simulink model "sus"  (Simulink 6.5)
settings: Solver=ode45  StartTime=0.0  StopTime=16  RelTol=1e-3
libraries: cdsFilt x266, cdsBitwise x92, cdsEpicsOut x84, cdsEpicsBinIn x56, cdsEpicsIn x20, cdsFiltCtrl x18, cdsMatrix x11, cdsSwitch x7, cdsWD x7, cdsFunctionCall x5, cdsRio1 x4, dac x3
(part 19 of 20)

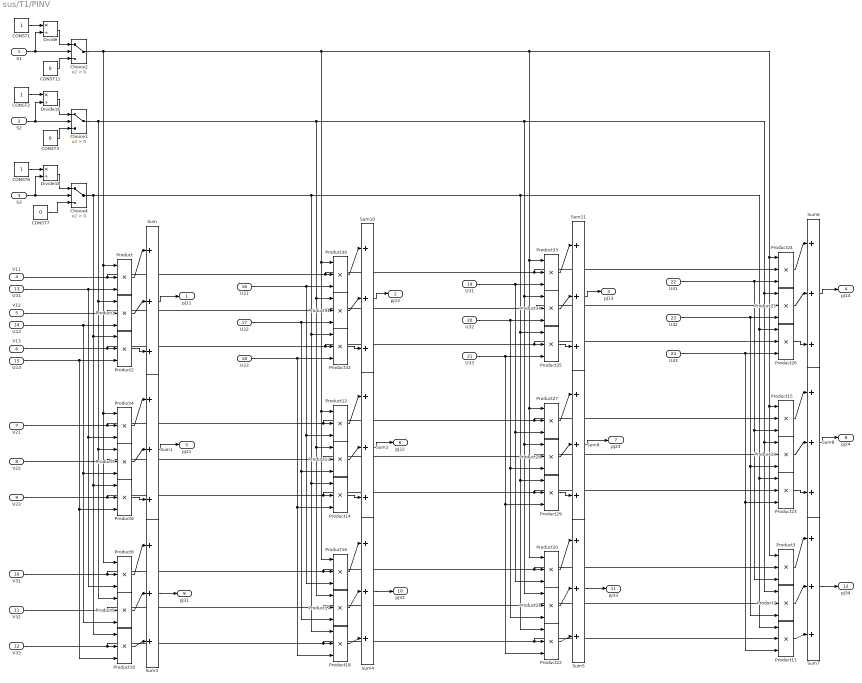
== system sus/T1/PINV ==
  S1 : Inport
  S2 : Inport  Port=2
  S3 : Inport  Port=3
  V11 : Inport  Port=4
  V12 : Inport  Port=5
  V13 : Inport  Port=6
  V21 : Inport  Port=7
  V22 : Inport  Port=8
  V23 : Inport  Port=9
  V31 : Inport  Port=10
  V32 : Inport  Port=11
  V33 : Inport  Port=12
  U11 : Inport  Port=13
  U12 : Inport  Port=14
  U13 : Inport  Port=15
  U21 : Inport  Port=16
  U22 : Inport  Port=17
  U23 : Inport  Port=18
  U31 : Inport  Port=19
  U32 : Inport  Port=20
  U33 : Inport  Port=21
  U41 : Inport  Port=22
  U42 : Inport  Port=23
  U43 : Inport  Port=24
  CONST1 : Constant
  CONST11 : Constant  Value=0
  CONST2 : Constant
  CONST3 : Constant  Value=0
  CONST6 : Constant
  CONST7 : Constant  Value=0
  Choice1 : Switch  Criteria=u2 > Threshold
  Choice2 : Switch  Criteria=u2 > Threshold
  Choice4 : Switch  Criteria=u2 > Threshold
  Divide : Product  Inputs=*/  OutScaling=2^-10
  Divide16 : Product  Inputs=*/  OutScaling=2^-10
  Divide18 : Product  Inputs=*/  OutScaling=2^-10
  Product{,1..35} (36 alike) : Product  Inputs=3  RndMeth=Zero
  Sum{,1..11} (12 alike) : Sum  Inputs=|+++
  pJ11 : Outport
  pJ12 : Outport  Port=2
  pJ13 : Outport  Port=3
  pJ14 : Outport  Port=4
  pJ21 : Outport  Port=5
  pJ22 : Outport  Port=6
  pJ23 : Outport  Port=7
  pJ24 : Outport  Port=8
  pJ31 : Outport  Port=9
  pJ32 : Outport  Port=10
  pJ33 : Outport  Port=11
  pJ34 : Outport  Port=12
  wires:
  Product/1 -> Sum/1
  S1/1 -> Choice2/2, Divide/2
  Divide/1 -> Choice2/1
  CONST11/1 -> Choice2/3
  CONST1/1 -> Divide/1
  Divide16/1 -> Choice1/1
  CONST3/1 -> Choice1/3
  CONST2/1 -> Divide16/1
  S2/1 -> Choice1/2, Divide16/2
  Divide18/1 -> Choice4/1
  CONST7/1 -> Choice4/3
  CONST6/1 -> Divide18/1
  S3/1 -> Choice4/2, Divide18/2
  Product1/1 -> Sum/2
  Product2/1 -> Sum/3
  Product4/1 -> Sum1/1
  Product5/1 -> Sum1/2
  Product6/1 -> Sum1/3
  Product8/1 -> Sum3/1
  Product9/1 -> Sum3/2
  Product10/1 -> Sum3/3
  Product30/1 -> Sum10/1
  Product31/1 -> Sum10/2
  Product32/1 -> Sum10/3
  Product12/1 -> Sum2/1
  Product13/1 -> Sum2/2
  Product14/1 -> Sum2/3
  Product16/1 -> Sum4/1
  Product17/1 -> Sum4/2
  Product18/1 -> Sum4/3
  Product33/1 -> Sum11/1
  Product34/1 -> Sum11/2
  Product35/1 -> Sum11/3
  Product27/1 -> Sum9/1
  Product28/1 -> Sum9/2
  Product29/1 -> Sum9/3
  Product20/1 -> Sum5/1
  Product21/1 -> Sum5/2
  Product22/1 -> Sum5/3
  Product24/1 -> Sum6/1
  Product25/1 -> Sum6/2
  Product26/1 -> Sum6/3
  Product15/1 -> Sum8/1
  Product19/1 -> Sum8/2
  Product23/1 -> Sum8/3
  Product3/1 -> Sum7/1
  Product7/1 -> Sum7/2
  Product11/1 -> Sum7/3
  Choice2/1 -> Product/1, Product4/1, Product8/1, Product33/1, Product20/1, Product27/1, Product24/1, Product3/1, Product15/1, Product30/1, Product12/1, Product16/1
  Choice1/1 -> Product1/1, Product5/1, Product9/1, Product34/1, Product21/1, Product28/1, Product25/1, Product7/1, Product19/1, Product31/1, Product17/1, Product13/1
  Choice4/1 -> Product2/1, Product6/1, Product10/1, Product35/1, Product22/1, Product29/1, Product26/1, Product11/1, Product23/1, Product32/1, Product18/1, Product14/1
  V11/1 -> Product/2, Product30/2, Product33/2, Product24/2
  U11/1 -> Product/3, Product4/3, Product8/3
  V12/1 -> Product1/2, Product31/2, Product34/2, Product25/2
  U12/1 -> Product1/3, Product5/3, Product9/3
  V13/1 -> Product2/2, Product32/2, Product35/2, Product26/2
  U13/1 -> Product2/3, Product6/3, Product10/3
  V21/1 -> Product4/2, Product12/2, Product27/2, Product15/2
  V22/1 -> Product5/2, Product13/2, Product28/2, Product19/2
  V23/1 -> Product6/2, Product14/2, Product29/2, Product23/2
  V31/1 -> Product8/2, Product16/2, Product20/2, Product3/2
  V32/1 -> Product9/2, Product17/2, Product21/2, Product7/2
  V33/1 -> Product10/2, Product18/2, Product22/2, Product11/2
  Sum/1 -> pJ11/1
  Sum1/1 -> pJ21/1
  Sum3/1 -> pJ31/1
  Sum10/1 -> pJ12/1
  Sum11/1 -> pJ13/1
  Sum6/1 -> pJ14/1
  Sum2/1 -> pJ22/1
  Sum9/1 -> pJ23/1
  Sum8/1 -> pJ24/1
  Sum4/1 -> pJ32/1
  Sum5/1 -> pJ33/1
  Sum7/1 -> pJ34/1
  U21/1 -> Product30/3, Product12/3, Product16/3
  U22/1 -> Product31/3, Product17/3, Product13/3
  U23/1 -> Product32/3, Product18/3, Product14/3
  U31/1 -> Product33/3, Product20/3, Product27/3
  U32/1 -> Product34/3, Product21/3, Product28/3
  U33/1 -> Product35/3, Product22/3, Product29/3
  U41/1 -> Product24/3, Product3/3, Product15/3
  U42/1 -> Product25/3, Product7/3, Product19/3
  U43/1 -> Product26/3, Product11/3, Product23/3

== system sus/T1/SQ1 ==
  11 : Inport
  12 : Inport  Port=2
  13 : Inport  Port=3
  21 : Inport  Port=4
  22 : Inport  Port=5
  23 : Inport  Port=6
  31 : Inport  Port=7
  32 : Inport  Port=8
  33 : Inport  Port=9
  41 : Inport  Port=10
  42 : Inport  Port=11
  43 : Inport  Port=12
  Product{,1..23} (24 alike) : Product  RndMeth=Zero
  Sum{,1..5} (6 alike) : Sum  Inputs=|++++
  Out11 : Outport
  Out12 : Outport  Port=2
  Out13 : Outport  Port=3
  Out21 : Outport  Port=4
  Out22 : Outport  Port=5
  Out23 : Outport  Port=6
  Out31 : Outport  Port=7
  Out32 : Outport  Port=8
  Out33 : Outport  Port=9
  wires:
  Product/1 -> Sum/1
  11/1 -> Product/1, Product/2, Product4/1, Product8/1
  Sum/1 -> Out11/1
  Product1/1 -> Sum/2
  Product2/1 -> Sum/3
  Product3/1 -> Sum/4
  21/1 -> Product1/1, Product1/2, Product5/1, Product9/1
  31/1 -> Product2/1, Product2/2, Product6/1, Product10/1
  41/1 -> Product3/1, Product3/2, Product7/1, Product11/1
  Product4/1 -> Sum1/1
  Product5/1 -> Sum1/2
  Product6/1 -> Sum1/3
  Product7/1 -> Sum1/4
  Sum1/1 -> Out21/1, Out12/1
  12/1 -> Product4/2, Product12/2, Product12/1, Product16/1
  22/1 -> Product5/2, Product13/2, Product13/1, Product17/1
  32/1 -> Product6/2, Product14/2, Product14/1, Product18/1
  42/1 -> Product7/2, Product15/2, Product15/1, Product19/1
  Product8/1 -> Sum2/1
  Product9/1 -> Sum2/2
  Product10/1 -> Sum2/3
  Product11/1 -> Sum2/4
  43/1 -> Product11/2, Product19/2, Product23/2, Product23/1
  33/1 -> Product10/2, Product18/2, Product22/2, Product22/1
  23/1 -> Product9/2, Product17/2, Product21/2, Product21/1
  13/1 -> Product8/2, Product16/2, Product20/2, Product20/1
  Sum2/1 -> Out31/1, Out13/1
  Product12/1 -> Sum3/1
  Product13/1 -> Sum3/2
  Product14/1 -> Sum3/3
  Product15/1 -> Sum3/4
  Sum3/1 -> Out22/1
  Product16/1 -> Sum4/1
  Product17/1 -> Sum4/2
  Product18/1 -> Sum4/3
  Product19/1 -> Sum4/4
  Sum4/1 -> Out32/1, Out23/1
  Product20/1 -> Sum5/1
  Product21/1 -> Sum5/2
  Product22/1 -> Sum5/3
  Product23/1 -> Sum5/4
  Sum5/1 -> Out33/1

== system sus/T1/SQRT_BOX ==
  In1 : Inport
  CONST11 : Constant  Value=0
  Choice : Switch  Threshold=1000
  Choice1 : Switch
  Choice2 : Switch  Threshold=1e10
  Choice3 : Switch  Threshold=0.01
  Choice4 : Switch  Threshold=1e-6
  Divide{,1..9} (10 alike) : Product  Inputs=*/  OutScaling=2^-10
  Gain : Gain  Gain=0.05
  Gain{1..10} (10 alike) : Gain  Gain=0.5
  Gain11 : Gain  Gain=0.0001
  Gain12 : Gain  Gain=0.000001
  Gain13 : Gain  Gain=100
  Gain14 : Gain  Gain=10000
  Sum{,1..9} (10 alike) : Sum  Inputs=|++
  Out1 : Outport
  wires:
  Divide/1 -> Sum/1
  Choice1/1 -> Choice/2, Choice2/2, Choice3/2, Choice4/2, Gain/1, Gain13/1, Gain14/1, Divide/1, Divide1/1, Divide2/1, Divide3/1, Divide4/1, Divide5/1, Divide6/1, Divide7/1, Divide8/1, Divide9/1, Gain12/1, Gain11/1
  Gain1/1 -> Sum1/2, Divide1/2
  Divide1/1 -> Sum1/1
  Sum1/1 -> Gain2/1
  Sum/1 -> Gain1/1
  Gain2/1 -> Sum2/2, Divide2/2
  Divide2/1 -> Sum2/1
  Sum2/1 -> Gain4/1
  Gain4/1 -> Sum3/2, Divide3/2
  Divide3/1 -> Sum3/1
  Sum3/1 -> Gain3/1
  Gain3/1 -> Sum4/2, Divide4/2
  Divide4/1 -> Sum4/1
  Sum4/1 -> Gain5/1
  Gain5/1 -> Sum5/2, Divide5/2
  Divide5/1 -> Sum5/1
  Sum5/1 -> Gain6/1
  Gain6/1 -> Sum6/2, Divide6/2
  Divide6/1 -> Sum6/1
  Sum6/1 -> Gain7/1
  Gain7/1 -> Sum7/2, Divide7/2
  Divide7/1 -> Sum7/1
  Sum7/1 -> Gain8/1
  Gain8/1 -> Sum8/2, Divide8/2
  Divide8/1 -> Sum8/1
  Sum8/1 -> Gain9/1
  Gain9/1 -> Sum9/2, Divide9/2
  Divide9/1 -> Sum9/1
  Sum9/1 -> Gain10/1
  Gain10/1 -> Out1/1
  Gain/1 -> Choice/3
  In1/1 -> Choice1/2, Choice1/1
  CONST11/1 -> Choice1/3
  Gain11/1 -> Choice2/3
  Gain12/1 -> Choice2/1
  Choice2/1 -> Choice/1
  Choice/1 -> Choice3/1
  Choice3/1 -> Choice4/1
  Choice4/1 -> Sum/2, Divide/2
  Gain13/1 -> Choice3/3
  Gain14/1 -> Choice4/3

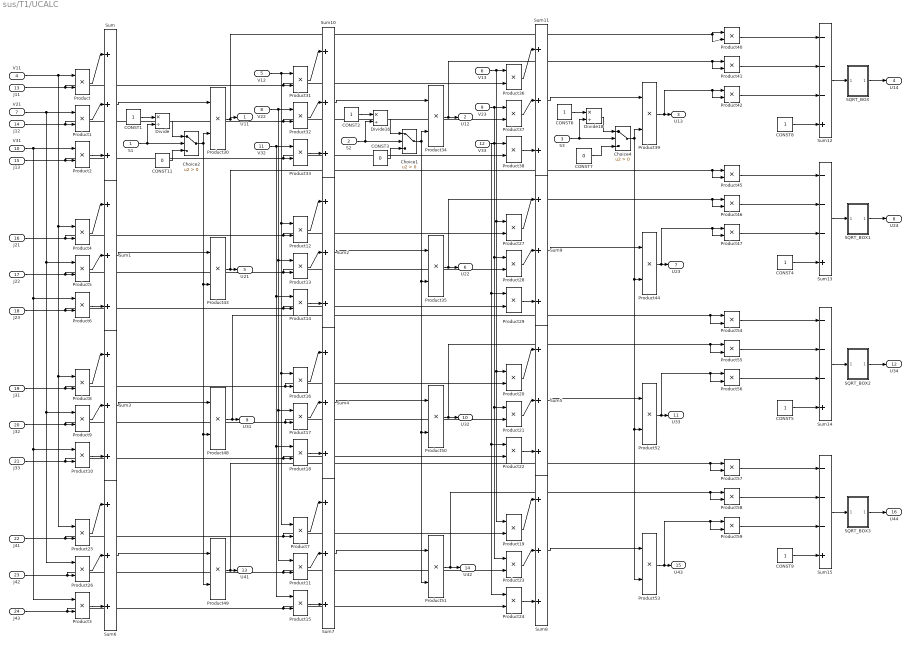
== system sus/T1/UCALC ==
  S1 : Inport
  S2 : Inport  Port=2
  S3 : Inport  Port=3
  V11 : Inport  Port=4
  V12 : Inport  Port=5
  V13 : Inport  Port=6
  V21 : Inport  Port=7
  V22 : Inport  Port=8
  V23 : Inport  Port=9
  V31 : Inport  Port=10
  V32 : Inport  Port=11
  V33 : Inport  Port=12
  J11 : Inport  Port=13
  J12 : Inport  Port=14
  J13 : Inport  Port=15
  J21 : Inport  Port=16
  J22 : Inport  Port=17
  J23 : Inport  Port=18
  J31 : Inport  Port=19
  J32 : Inport  Port=20
  J33 : Inport  Port=21
  J41 : Inport  Port=22
  J42 : Inport  Port=23
  J43 : Inport  Port=24
  CONST{1..2,4..6,8..9} (7 alike) : Constant
  CONST11 : Constant  Value=0
  CONST3 : Constant  Value=0
  CONST7 : Constant  Value=0
  Choice1 : Switch  Criteria=u2 > Threshold
  Choice2 : Switch  Criteria=u2 > Threshold
  Choice4 : Switch  Criteria=u2 > Threshold
  Divide : Product  Inputs=*/  OutScaling=2^-10
  Divide16 : Product  Inputs=*/  OutScaling=2^-10
  Divide18 : Product  Inputs=*/  OutScaling=2^-10
  Product{,1..59} (60 alike) : Product  RndMeth=Zero
  SQRT_BOX : Subsystem
  SQRT_BOX1 : Subsystem
  SQRT_BOX2 : Subsystem
  SQRT_BOX3 : Subsystem
  Sum{,1..11} (12 alike) : Sum  Inputs=|+++
  Sum{12..15} (4 alike) : Sum  Inputs=---+
  U11 : Outport
  U12 : Outport  Port=2
  U13 : Outport  Port=3
  U14 : Outport  Port=4
  U21 : Outport  Port=5
  U22 : Outport  Port=6
  U23 : Outport  Port=7
  U24 : Outport  Port=8
  U31 : Outport  Port=9
  U32 : Outport  Port=10
  U33 : Outport  Port=11
  U34 : Outport  Port=12
  U41 : Outport  Port=13
  U42 : Outport  Port=14
  U43 : Outport  Port=15
  U44 : Outport  Port=16
  wires:
  Product20/1 -> Sum5/1
  Product21/1 -> Sum5/2
  Product22/1 -> Sum5/3
  Product19/1 -> Sum8/1
  Product23/1 -> Sum8/2
  Product24/1 -> Sum8/3
  Product12/1 -> Sum2/1
  Product13/1 -> Sum2/2
  Product14/1 -> Sum2/3
  Product16/1 -> Sum4/1
  Product17/1 -> Sum4/2
  Product18/1 -> Sum4/3
  Product7/1 -> Sum7/1
  Product11/1 -> Sum7/2
  Product15/1 -> Sum7/3
  Product/1 -> Sum/1
  Product1/1 -> Sum/2
  Product2/1 -> Sum/3
  Product4/1 -> Sum1/1
  Product5/1 -> Sum1/2
  Product6/1 -> Sum1/3
  Product8/1 -> Sum3/1
  Product9/1 -> Sum3/2
  Product10/1 -> Sum3/3
  Product25/1 -> Sum6/1
  Product26/1 -> Sum6/2
  Product3/1 -> Sum6/3
  V11/1 -> Product/1, Product4/1, Product8/1, Product25/1
  J11/1 -> Product/2, Product31/2, Product36/2
  V21/1 -> Product1/1, Product5/1, Product9/1, Product26/1
  J12/1 -> Product1/2, Product32/2, Product37/2
  J13/1 -> Product2/2, Product33/2, Product38/2
  V31/1 -> Product2/1, Product6/1, Product10/1, Product3/1
  S1/1 -> Choice2/2, Divide/2
  Divide/1 -> Choice2/1
  CONST11/1 -> Choice2/3
  CONST1/1 -> Divide/1
  Product30/1 -> U11/1, Product40/1, Product40/2
  Choice2/1 -> Product30/2, Product43/2, Product48/2, Product49/2
  Sum/1 -> Product30/1
  Product31/1 -> Sum10/1
  Product32/1 -> Sum10/2
  Product33/1 -> Sum10/3
  V12/1 -> Product31/1, Product12/1, Product16/1, Product7/1
  V22/1 -> Product32/1, Product13/1, Product17/1, Product11/1
  V32/1 -> Product33/1, Product14/1, Product18/1, Product15/1
  Divide16/1 -> Choice1/1
  CONST3/1 -> Choice1/3
  CONST2/1 -> Divide16/1
  Choice1/1 -> Product34/2, Product35/2, Product50/2, Product51/2
  Sum10/1 -> Product34/1
  S2/1 -> Choice1/2, Divide16/2
  Product34/1 -> U12/1, Product41/1, Product41/2
  Product36/1 -> Sum11/1
  Product37/1 -> Sum11/2
  Product38/1 -> Sum11/3
  V13/1 -> Product36/1, Product27/1, Product20/1, Product19/1
  V23/1 -> Product37/1, Product28/1, Product21/1, Product23/1
  V33/1 -> Product38/1, Product29/1, Product22/1, Product24/1
  Divide18/1 -> Choice4/1
  CONST7/1 -> Choice4/3
  CONST6/1 -> Divide18/1
  Choice4/1 -> Product39/2, Product44/2, Product52/2, Product53/2
  Sum11/1 -> Product39/1
  S3/1 -> Choice4/2, Divide18/2
  Product39/1 -> U13/1, Product42/1, Product42/2
  J21/1 -> Product4/2, Product12/2, Product27/2
  J22/1 -> Product5/2, Product13/2, Product28/2
  J23/1 -> Product6/2, Product14/2, Product29/2
  J31/1 -> Product8/2, Product16/2, Product20/2
  J32/1 -> Product9/2, Product17/2, Product21/2
  J33/1 -> Product10/2, Product18/2, Product22/2
  J41/1 -> Product25/2, Product7/2, Product19/2
  J42/1 -> Product26/2, Product11/2, Product23/2
  J43/1 -> Product3/2, Product15/2, Product24/2
  CONST8/1 -> Sum12/4
  Product40/1 -> Sum12/1
  Product41/1 -> Sum12/2
  Product42/1 -> Sum12/3
  Sum12/1 -> SQRT_BOX/1(In1)
  SQRT_BOX/1(Out1) -> U14/1
  Product27/1 -> Sum9/1
  Product28/1 -> Sum9/2
  Sum1/1 -> Product43/1
  Product43/1 -> U21/1, Product45/1, Product45/2
  Sum2/1 -> Product35/1
  Product35/1 -> U22/1, Product46/1, Product46/2
  Sum9/1 -> Product44/1
  Product44/1 -> U23/1, Product47/1, Product47/2
  CONST4/1 -> Sum13/4
  Product45/1 -> Sum13/1
  Product46/1 -> Sum13/2
  Product47/1 -> Sum13/3
  Sum13/1 -> SQRT_BOX1/1(In1)
  SQRT_BOX1/1(Out1) -> U24/1
  Sum3/1 -> Product48/1
  Product48/1 -> U31/1, Product54/1, Product54/2
  Sum6/1 -> Product49/1
  Product49/1 -> U41/1, Product57/1, Product57/2
  Product50/1 -> U32/1, Product55/1, Product55/2
  Product51/1 -> U42/1, Product58/1, Product58/2
  Sum4/1 -> Product50/1
  Sum7/1 -> Product51/1
  Sum5/1 -> Product52/1
  Product52/1 -> U33/1, Product56/1, Product56/2
  Product53/1 -> U43/1, Product59/1, Product59/2
  Sum8/1 -> Product53/1
  CONST5/1 -> Sum14/4
  Product54/1 -> Sum14/1
  Product55/1 -> Sum14/2
  Product56/1 -> Sum14/3
  Sum14/1 -> SQRT_BOX2/1(In1)
  SQRT_BOX2/1(Out1) -> U34/1
  CONST9/1 -> Sum15/4
  Product57/1 -> Sum15/1
  Product58/1 -> Sum15/2
  Product59/1 -> Sum15/3
  Sum15/1 -> SQRT_BOX3/1(In1)
  SQRT_BOX3/1(Out1) -> U44/1
  Product29/1 -> Sum9/3

== system sus/T1/VECNORM ==
  3311 : Inport
  3312 : Inport  Port=2
  3313 : Inport  Port=3
  3321 : Inport  Port=4
  3322 : Inport  Port=5
  3323 : Inport  Port=6
  3331 : Inport  Port=7
  3332 : Inport  Port=8
  3333 : Inport  Port=9
  Divide{,1..8} (9 alike) : Product  Inputs=*/  OutScaling=2^-10
  Product{1..9} (9 alike) : Product  RndMeth=Zero
  SQRT_BOX1 : Subsystem
  SQRT_BOX2 : Subsystem
  SQRT_BOX3 : Subsystem
  Sum1 : Sum  Inputs=+++
  Sum2 : Sum  Inputs=+++
  Sum8 : Sum  Inputs=+++
  Out3311 : Outport
  Out3312 : Outport  Port=2
  Out3313 : Outport  Port=3
  Out3321 : Outport  Port=4
  Out3322 : Outport  Port=5
  Out3323 : Outport  Port=6
  Out3331 : Outport  Port=7
  Out3332 : Outport  Port=8
  Out3333 : Outport  Port=9
  wires:
  Divide8/1 -> Out3333/1
  Divide7/1 -> Out3323/1
  SQRT_BOX3/1(Out1) -> Divide8/2, Divide7/2, Divide6/2
  Divide6/1 -> Out3313/1
  Sum2/1 -> SQRT_BOX3/1(In1)
  Product8/1 -> Sum2/3
  Product7/1 -> Sum2/2
  Product9/1 -> Sum2/1
  3333/1 -> Divide8/1, Product8/1, Product8/2
  3323/1 -> Divide7/1, Product7/2, Product7/1
  3313/1 -> Divide6/1, Product9/2, Product9/1
  Divide5/1 -> Out3332/1
  Divide4/1 -> Out3322/1
  SQRT_BOX2/1(Out1) -> Divide5/2, Divide4/2, Divide3/2
  Divide3/1 -> Out3312/1
  Sum1/1 -> SQRT_BOX2/1(In1)
  Product4/1 -> Sum1/3
  Product2/1 -> Sum1/2
  Product5/1 -> Sum1/1
  3332/1 -> Divide5/1, Product4/1, Product4/2
  3322/1 -> Divide4/1, Product2/2, Product2/1
  3312/1 -> Divide3/1, Product5/2, Product5/1
  Divide2/1 -> Out3331/1
  Divide1/1 -> Out3321/1
  SQRT_BOX1/1(Out1) -> Divide2/2, Divide1/2, Divide/2
  Divide/1 -> Out3311/1
  Sum8/1 -> SQRT_BOX1/1(In1)
  Product3/1 -> Sum8/3
  Product1/1 -> Sum8/2
  Product6/1 -> Sum8/1
  3331/1 -> Divide2/1, Product3/1, Product3/2
  3321/1 -> Divide1/1, Product1/2, Product1/1
  3311/1 -> Divide/1, Product6/2, Product6/1

== system sus/Q1/M0/ADD ==
  In1 : Inport
  In2 : Inport  Port=2
  In3 : Inport  Port=3
  In4 : Inport  Port=4
  In5 : Inport  Port=5
  In6 : Inport  Port=6
  In7 : Inport  Port=7
  In8 : Inport  Port=8
  In9 : Inport  Port=9
  In10 : Inport  Port=10
  In11 : Inport  Port=11
  In12 : Inport  Port=12
  Sum{,1..5} (6 alike) : Sum  Inputs=|++
  Out1 : Outport
  Out2 : Outport  Port=2
  Out3 : Outport  Port=3
  Out4 : Outport  Port=4
  Out5 : Outport  Port=5
  Out6 : Outport  Port=6
  wires:
  In1/1 -> Sum/1
  Sum/1 -> Out1/1
  Sum1/1 -> Out2/1
  In2/1 -> Sum1/1
  In3/1 -> Sum2/1
  Sum2/1 -> Out3/1
  Sum3/1 -> Out4/1
  In4/1 -> Sum3/1
  In5/1 -> Sum4/1
  Sum4/1 -> Out5/1
  Sum5/1 -> Out6/1
  In6/1 -> Sum5/1
  In7/1 -> Sum/2
  In8/1 -> Sum1/2
  In9/1 -> Sum2/2
  In10/1 -> Sum3/2
  In11/1 -> Sum4/2
  In12/1 -> Sum5/2

== system sus/Q1/M0/BIT ==
  In1 : Inport
  In3 : Inport  Port=2
  In2 : Inport  Port=3
  In4 : Inport  Port=4
  In5 : Inport  Port=5
  In6 : Inport  Port=6
  Constant1 : Constant  Value=4
  Constant2 : Constant  Value=0
  Constant6 : Constant  Value=67108864
  Constant8 : Constant  Value=0
  LogicalOperator10 : Logic  Inputs=12  AllPortsSameDT=off  OutDataTypeMode=Boolean
  Operator{1..12} (12 alike) : RelationalOperator  Operator=~=  LogicOutDataTypeMode=Boolean
  and{1..12} (12 alike) : cdsBitwise/Subsystem  Tag=cdsBitwise  SystemSampleTime=-1
      settings: AttributesFormatString=%<Tag>
  Out1 : Outport
  wires:
  and1/1 -> Operator4/1
  Constant8/1 -> Operator6/2, Operator4/2, Operator1/2, Operator2/2, Operator3/2, Operator5/2
  and4/1 -> Operator1/1
  In1/1 -> and4/1, and10/1
  In3/1 -> and1/1, and7/1
  and2/1 -> Operator2/1
  In2/1 -> and2/1, and8/1
  and3/1 -> Operator3/1
  In4/1 -> and3/1, and9/1
  and5/1 -> Operator5/1
  In5/1 -> and5/1, and11/1
  and6/1 -> Operator6/1
  In6/1 -> and6/1, and12/1
  Constant6/1 -> and4/2, and1/2, and2/2, and3/2, and5/2, and6/2
  and7/1 -> Operator10/1
  Constant2/1 -> Operator12/2, Operator10/2, Operator7/2, Operator8/2, Operator9/2, Operator11/2
  and10/1 -> Operator7/1
  and8/1 -> Operator8/1
  and9/1 -> Operator9/1
  and11/1 -> Operator11/1
  and12/1 -> Operator12/1
  Constant1/1 -> and10/2, and7/2, and8/2, and9/2, and11/2, and12/2
  LogicalOperator10/1 -> Out1/1
  Operator1/1 -> LogicalOperator10/1
  Operator4/1 -> LogicalOperator10/2
  Operator2/1 -> LogicalOperator10/3
  Operator3/1 -> LogicalOperator10/4
  Operator5/1 -> LogicalOperator10/5
  Operator6/1 -> LogicalOperator10/6
  Operator7/1 -> LogicalOperator10/7
  Operator10/1 -> LogicalOperator10/8
  Operator8/1 -> LogicalOperator10/9
  Operator9/1 -> LogicalOperator10/10
  Operator11/1 -> LogicalOperator10/11
  Operator12/1 -> LogicalOperator10/12

== system sus/Q1/R0/ADD ==
  In1 : Inport
  In2 : Inport  Port=2
  In3 : Inport  Port=3
  In4 : Inport  Port=4
  In5 : Inport  Port=5
  In6 : Inport  Port=6
  In7 : Inport  Port=7
  In8 : Inport  Port=8
  In9 : Inport  Port=9
  In10 : Inport  Port=10
  In11 : Inport  Port=11
  In12 : Inport  Port=12
  Sum{,1..5} (6 alike) : Sum  Inputs=|++
  Out1 : Outport
  Out2 : Outport  Port=2
  Out3 : Outport  Port=3
  Out4 : Outport  Port=4
  Out5 : Outport  Port=5
  Out6 : Outport  Port=6
  wires:
  In1/1 -> Sum/1
  Sum/1 -> Out1/1
  Sum1/1 -> Out2/1
  In2/1 -> Sum1/1
  In3/1 -> Sum2/1
  Sum2/1 -> Out3/1
  Sum3/1 -> Out4/1
  In4/1 -> Sum3/1
  In5/1 -> Sum4/1
  Sum4/1 -> Out5/1
  Sum5/1 -> Out6/1
  In6/1 -> Sum5/1
  In7/1 -> Sum/2
  In8/1 -> Sum1/2
  In9/1 -> Sum2/2
  In10/1 -> Sum3/2
  In11/1 -> Sum4/2
  In12/1 -> Sum5/2

== system sus/Q1/R0/BIT ==
  In1 : Inport
  In3 : Inport  Port=2
  In2 : Inport  Port=3
  In4 : Inport  Port=4
  In5 : Inport  Port=5
  In6 : Inport  Port=6
  Constant1 : Constant  Value=4
  Constant2 : Constant  Value=0
  Constant6 : Constant  Value=67108864
  Constant8 : Constant  Value=0
  LogicalOperator10 : Logic  Inputs=12  AllPortsSameDT=off  OutDataTypeMode=Boolean
  Operator{1..12} (12 alike) : RelationalOperator  Operator=~=  LogicOutDataTypeMode=Boolean
  and{1..12} (12 alike) : cdsBitwise/Subsystem  Tag=cdsBitwise  SystemSampleTime=-1
      settings: AttributesFormatString=%<Tag>
  Out1 : Outport
  wires:
  and1/1 -> Operator4/1
  Constant8/1 -> Operator6/2, Operator4/2, Operator1/2, Operator2/2, Operator3/2, Operator5/2
  and4/1 -> Operator1/1
  In1/1 -> and4/1, and10/1
  In3/1 -> and1/1, and7/1
  and2/1 -> Operator2/1
  In2/1 -> and2/1, and8/1
  and3/1 -> Operator3/1
  In4/1 -> and3/1, and9/1
  and5/1 -> Operator5/1
  In5/1 -> and5/1, and11/1
  and6/1 -> Operator6/1
  In6/1 -> and6/1, and12/1
  Constant6/1 -> and4/2, and1/2, and2/2, and3/2, and5/2, and6/2
  and7/1 -> Operator10/1
  Constant2/1 -> Operator12/2, Operator10/2, Operator7/2, Operator8/2, Operator9/2, Operator11/2
  and10/1 -> Operator7/1
  and8/1 -> Operator8/1
  and9/1 -> Operator9/1
  and11/1 -> Operator11/1
  and12/1 -> Operator12/1
  Constant1/1 -> and10/2, and7/2, and8/2, and9/2, and11/2, and12/2
  LogicalOperator10/1 -> Out1/1
  Operator1/1 -> LogicalOperator10/1
  Operator4/1 -> LogicalOperator10/2
  Operator2/1 -> LogicalOperator10/3
  Operator3/1 -> LogicalOperator10/4
  Operator5/1 -> LogicalOperator10/5
  Operator6/1 -> LogicalOperator10/6
  Operator7/1 -> LogicalOperator10/7
  Operator10/1 -> LogicalOperator10/8
  Operator8/1 -> LogicalOperator10/9
  Operator9/1 -> LogicalOperator10/10
  Operator11/1 -> LogicalOperator10/11
  Operator12/1 -> LogicalOperator10/12

== system sus/RLS/DELTA1/HOLD ==
  In1 : Inport
  time : Inport  Port=2
  delay_in : Inport  Port=3
  CONST1 : Constant  Value=0
  CONST2 : Constant  Value=0
  Choice1 : Switch  Threshold=0.5-(1/16384)
  Choice2 : Switch  Threshold=0.5-(1/16384)
  Gain1 : Gain
  Gain2 : Gain  Gain=-1
  Sum8 : Sum  Inputs=+++
  out : Outport
  delay_out : Outport  Port=2
  wires:
  CONST2/1 -> Choice2/3
  time/1 -> Choice2/2, Choice1/2
  In1/1 -> Choice2/1
  Choice2/1 -> Sum8/2
  Sum8/1 -> delay_out/1
  delay_in/1 -> Gain2/1, Sum8/3, Gain1/1
  CONST1/1 -> Choice1/3
  Gain2/1 -> Choice1/1
  Choice1/1 -> Sum8/1
  Gain1/1 -> out/1

== system sus/RLS/DELTA2/HOLD ==
  In1 : Inport
  time : Inport  Port=2
  delay_in : Inport  Port=3
  CONST1 : Constant  Value=0
  CONST2 : Constant  Value=0
  Choice1 : Switch  Threshold=0.5-(1/16384)
  Choice2 : Switch  Threshold=0.5-(1/16384)
  Gain1 : Gain
  Gain2 : Gain  Gain=-1
  Sum8 : Sum  Inputs=+++
  out : Outport
  delay_out : Outport  Port=2
  wires:
  CONST2/1 -> Choice2/3
  time/1 -> Choice2/2, Choice1/2
  In1/1 -> Choice2/1
  Choice2/1 -> Sum8/2
  Sum8/1 -> delay_out/1
  delay_in/1 -> Gain2/1, Sum8/3, Gain1/1
  CONST1/1 -> Choice1/3
  Gain2/1 -> Choice1/1
  Choice1/1 -> Sum8/1
  Gain1/1 -> out/1

== system sus/RLS/DELTA3/HOLD ==
  In1 : Inport
  time : Inport  Port=2
  delay_in : Inport  Port=3
  CONST1 : Constant  Value=0
  CONST2 : Constant  Value=0
  Choice1 : Switch  Threshold=0.5-(1/16384)
  Choice2 : Switch  Threshold=0.5-(1/16384)
  Gain1 : Gain
  Gain2 : Gain  Gain=-1
  Sum8 : Sum  Inputs=+++
  out : Outport
  delay_out : Outport  Port=2
  wires:
  CONST2/1 -> Choice2/3
  time/1 -> Choice2/2, Choice1/2
  In1/1 -> Choice2/1
  Choice2/1 -> Sum8/2
  Sum8/1 -> delay_out/1
  delay_in/1 -> Gain2/1, Sum8/3, Gain1/1
  CONST1/1 -> Choice1/3
  Gain2/1 -> Choice1/1
  Choice1/1 -> Sum8/1
  Gain1/1 -> out/1

== system sus/RLS/J11/HOLD ==
  In1 : Inport
  time : Inport  Port=2
  delay_in : Inport  Port=3
  CONST1 : Constant  Value=0
  CONST2 : Constant  Value=0
  Choice1 : Switch  Threshold=0.5-(1/16384)
  Choice2 : Switch  Threshold=0.5-(1/16384)
  Gain1 : Gain
  Gain2 : Gain  Gain=-1
  Sum8 : Sum  Inputs=+++
  out : Outport
  delay_out : Outport  Port=2
  wires:
  CONST2/1 -> Choice2/3
  time/1 -> Choice2/2, Choice1/2
  In1/1 -> Choice2/1
  Choice2/1 -> Sum8/2
  Sum8/1 -> delay_out/1
  delay_in/1 -> Gain2/1, Sum8/3, Gain1/1
  CONST1/1 -> Choice1/3
  Gain2/1 -> Choice1/1
  Choice1/1 -> Sum8/1
  Gain1/1 -> out/1

== system sus/RLS/J12/HOLD ==
  In1 : Inport
  time : Inport  Port=2
  delay_in : Inport  Port=3
  CONST1 : Constant  Value=0
  CONST2 : Constant  Value=0
  Choice1 : Switch  Threshold=0.5-(1/16384)
  Choice2 : Switch  Threshold=0.5-(1/16384)
  Gain1 : Gain
  Gain2 : Gain  Gain=-1
  Sum8 : Sum  Inputs=+++
  out : Outport
  delay_out : Outport  Port=2
  wires:
  CONST2/1 -> Choice2/3
  time/1 -> Choice2/2, Choice1/2
  In1/1 -> Choice2/1
  Choice2/1 -> Sum8/2
  Sum8/1 -> delay_out/1
  delay_in/1 -> Gain2/1, Sum8/3, Gain1/1
  CONST1/1 -> Choice1/3
  Gain2/1 -> Choice1/1
  Choice1/1 -> Sum8/1
  Gain1/1 -> out/1

== system sus/RLS/J21/HOLD ==
  In1 : Inport
  time : Inport  Port=2
  delay_in : Inport  Port=3
  CONST1 : Constant  Value=0
  CONST2 : Constant  Value=0
  Choice1 : Switch  Threshold=0.5-(1/16384)
  Choice2 : Switch  Threshold=0.5-(1/16384)
  Gain1 : Gain
  Gain2 : Gain  Gain=-1
  Sum8 : Sum  Inputs=+++
  out : Outport
  delay_out : Outport  Port=2
  wires:
  CONST2/1 -> Choice2/3
  time/1 -> Choice2/2, Choice1/2
  In1/1 -> Choice2/1
  Choice2/1 -> Sum8/2
  Sum8/1 -> delay_out/1
  delay_in/1 -> Gain2/1, Sum8/3, Gain1/1
  CONST1/1 -> Choice1/3
  Gain2/1 -> Choice1/1
  Choice1/1 -> Sum8/1
  Gain1/1 -> out/1

== system sus/RLS/J22/HOLD ==
  In1 : Inport
  time : Inport  Port=2
  delay_in : Inport  Port=3
  CONST1 : Constant  Value=0
  CONST2 : Constant  Value=0
  Choice1 : Switch  Threshold=0.5-(1/16384)
  Choice2 : Switch  Threshold=0.5-(1/16384)
  Gain1 : Gain
  Gain2 : Gain  Gain=-1
  Sum8 : Sum  Inputs=+++
  out : Outport
  delay_out : Outport  Port=2
  wires:
  CONST2/1 -> Choice2/3
  time/1 -> Choice2/2, Choice1/2
  In1/1 -> Choice2/1
  Choice2/1 -> Sum8/2
  Sum8/1 -> delay_out/1
  delay_in/1 -> Gain2/1, Sum8/3, Gain1/1
  CONST1/1 -> Choice1/3
  Gain2/1 -> Choice1/1
  Choice1/1 -> Sum8/1
  Gain1/1 -> out/1

== system sus/RLS/J31/HOLD ==
  In1 : Inport
  time : Inport  Port=2
  delay_in : Inport  Port=3
  CONST1 : Constant  Value=0
  CONST2 : Constant  Value=0
  Choice1 : Switch  Threshold=0.5-(1/16384)
  Choice2 : Switch  Threshold=0.5-(1/16384)
  Gain1 : Gain
  Gain2 : Gain  Gain=-1
  Sum8 : Sum  Inputs=+++
  out : Outport
  delay_out : Outport  Port=2
  wires:
  CONST2/1 -> Choice2/3
  time/1 -> Choice2/2, Choice1/2
  In1/1 -> Choice2/1
  Choice2/1 -> Sum8/2
  Sum8/1 -> delay_out/1
  delay_in/1 -> Gain2/1, Sum8/3, Gain1/1
  CONST1/1 -> Choice1/3
  Gain2/1 -> Choice1/1
  Choice1/1 -> Sum8/1
  Gain1/1 -> out/1

== system sus/RLS/J32/HOLD ==
  In1 : Inport
  time : Inport  Port=2
  delay_in : Inport  Port=3
  CONST1 : Constant  Value=0
  CONST2 : Constant  Value=0
  Choice1 : Switch  Threshold=0.5-(1/16384)
  Choice2 : Switch  Threshold=0.5-(1/16384)
  Gain1 : Gain
  Gain2 : Gain  Gain=-1
  Sum8 : Sum  Inputs=+++
  out : Outport
  delay_out : Outport  Port=2
  wires:
  CONST2/1 -> Choice2/3
  time/1 -> Choice2/2, Choice1/2
  In1/1 -> Choice2/1
  Choice2/1 -> Sum8/2
  Sum8/1 -> delay_out/1
  delay_in/1 -> Gain2/1, Sum8/3, Gain1/1
  CONST1/1 -> Choice1/3
  Gain2/1 -> Choice1/1
  Choice1/1 -> Sum8/1
  Gain1/1 -> out/1

== system sus/RLS/K1/PDTHETA ==
  P11 : Inport
  P12 : Inport  Port=2
  P21 : Inport  Port=3
  P22 : Inport  Port=4
  dtheta1 : Inport  Port=5
  dtheta2 : Inport  Port=6
  Product{,1..3} (4 alike) : Product  RndMeth=Zero
  Sum : Sum  Inputs=|++
  Sum1 : Sum  Inputs=|++
  out1 : Outport
  out2 : Outport  Port=2
  wires:
  Product/1 -> Sum/1
  Sum/1 -> out1/1
  Product1/1 -> Sum/2
  Product2/1 -> Sum1/1
  Sum1/1 -> out2/1
  Product3/1 -> Sum1/2
  dtheta1/1 -> Product/1, Product2/1
  dtheta2/1 -> Product1/1, Product3/1
  P11/1 -> Product/2
  P12/1 -> Product1/2
  P21/1 -> Product2/2
  P22/1 -> Product3/2

== system sus/RLS/K2/PDTHETA ==
  P11 : Inport
  P12 : Inport  Port=2
  P21 : Inport  Port=3
  P22 : Inport  Port=4
  dtheta1 : Inport  Port=5
  dtheta2 : Inport  Port=6
  Product{,1..3} (4 alike) : Product  RndMeth=Zero
  Sum : Sum  Inputs=|++
  Sum1 : Sum  Inputs=|++
  out1 : Outport
  out2 : Outport  Port=2
  wires:
  Product/1 -> Sum/1
  Sum/1 -> out1/1
  Product1/1 -> Sum/2
  Product2/1 -> Sum1/1
  Sum1/1 -> out2/1
  Product3/1 -> Sum1/2
  dtheta1/1 -> Product/1, Product2/1
  dtheta2/1 -> Product1/1, Product3/1
  P11/1 -> Product/2
  P12/1 -> Product1/2
  P21/1 -> Product2/2
  P22/1 -> Product3/2

== system sus/RLS/K3/PDTHETA ==
  P11 : Inport
  P12 : Inport  Port=2
  P21 : Inport  Port=3
  P22 : Inport  Port=4
  dtheta1 : Inport  Port=5
  dtheta2 : Inport  Port=6
  Product{,1..3} (4 alike) : Product  RndMeth=Zero
  Sum : Sum  Inputs=|++
  Sum1 : Sum  Inputs=|++
  out1 : Outport
  out2 : Outport  Port=2
  wires:
  Product/1 -> Sum/1
  Sum/1 -> out1/1
  Product1/1 -> Sum/2
  Product2/1 -> Sum1/1
  Sum1/1 -> out2/1
  Product3/1 -> Sum1/2
  dtheta1/1 -> Product/1, Product2/1
  dtheta2/1 -> Product1/1, Product3/1
  P11/1 -> Product/2
  P12/1 -> Product1/2
  P21/1 -> Product2/2
  P22/1 -> Product3/2

== system sus/RLS/P1/HOLD ==
  In1 : Inport
  time : Inport  Port=2
  delay_in : Inport  Port=3
  CONST1 : Constant  Value=0
  CONST2 : Constant  Value=0
  Choice1 : Switch  Threshold=0.5-(1/16384)
  Choice2 : Switch  Threshold=0.5-(1/16384)
  Gain1 : Gain
  Gain2 : Gain  Gain=-1
  Sum8 : Sum  Inputs=+++
  out : Outport
  delay_out : Outport  Port=2
  wires:
  CONST2/1 -> Choice2/3
  time/1 -> Choice2/2, Choice1/2
  In1/1 -> Choice2/1
  Choice2/1 -> Sum8/2
  Sum8/1 -> delay_out/1
  delay_in/1 -> Gain2/1, Sum8/3, Gain1/1
  CONST1/1 -> Choice1/3
  Gain2/1 -> Choice1/1
  Choice1/1 -> Sum8/1
  Gain1/1 -> out/1

== system sus/RLS/P1/HOLD1 ==
  In1 : Inport
  time : Inport  Port=2
  delay_in : Inport  Port=3
  CONST1 : Constant  Value=0
  CONST2 : Constant  Value=0
  Choice1 : Switch  Threshold=0.5-(1/16384)
  Choice2 : Switch  Threshold=0.5-(1/16384)
  Gain1 : Gain
  Gain2 : Gain  Gain=-1
  Sum8 : Sum  Inputs=+++
  out : Outport
  delay_out : Outport  Port=2
  wires:
  CONST2/1 -> Choice2/3
  time/1 -> Choice2/2, Choice1/2
  In1/1 -> Choice2/1
  Choice2/1 -> Sum8/2
  Sum8/1 -> delay_out/1
  delay_in/1 -> Gain2/1, Sum8/3, Gain1/1
  CONST1/1 -> Choice1/3
  Gain2/1 -> Choice1/1
  Choice1/1 -> Sum8/1
  Gain1/1 -> out/1

== system sus/RLS/P1/HOLD2 ==
  In1 : Inport
  time : Inport  Port=2
  delay_in : Inport  Port=3
  CONST1 : Constant  Value=0
  CONST2 : Constant  Value=0
  Choice1 : Switch  Threshold=0.5-(1/16384)
  Choice2 : Switch  Threshold=0.5-(1/16384)
  Gain1 : Gain
  Gain2 : Gain  Gain=-1
  Sum8 : Sum  Inputs=+++
  out : Outport
  delay_out : Outport  Port=2
  wires:
  CONST2/1 -> Choice2/3
  time/1 -> Choice2/2, Choice1/2
  In1/1 -> Choice2/1
  Choice2/1 -> Sum8/2
  Sum8/1 -> delay_out/1
  delay_in/1 -> Gain2/1, Sum8/3, Gain1/1
  CONST1/1 -> Choice1/3
  Gain2/1 -> Choice1/1
  Choice1/1 -> Sum8/1
  Gain1/1 -> out/1

== system sus/RLS/P1/HOLD3 ==
  In1 : Inport
  time : Inport  Port=2
  delay_in : Inport  Port=3
  CONST1 : Constant  Value=0
  CONST2 : Constant  Value=0
  Choice1 : Switch  Threshold=0.5-(1/16384)
  Choice2 : Switch  Threshold=0.5-(1/16384)
  Gain1 : Gain
  Gain2 : Gain  Gain=-1
  Sum8 : Sum  Inputs=+++
  out : Outport
  delay_out : Outport  Port=2
  wires:
  CONST2/1 -> Choice2/3
  time/1 -> Choice2/2, Choice1/2
  In1/1 -> Choice2/1
  Choice2/1 -> Sum8/2
  Sum8/1 -> delay_out/1
  delay_in/1 -> Gain2/1, Sum8/3, Gain1/1
  CONST1/1 -> Choice1/3
  Gain2/1 -> Choice1/1
  Choice1/1 -> Sum8/1
  Gain1/1 -> out/1

== system sus/RLS/P1/MATH ==
  note: I - K*dtheta'
  K1_1 : Inport
  K1_2 : Inport  Port=2
  dtheta1 : Inport  Port=3
  dtheta2 : Inport  Port=4
  Gain1 : Gain  Gain=-1
  Gain2 : Gain  Gain=-1
  Product{,1..3} (4 alike) : Product  RndMeth=Zero
  SR : Constant
  Sum : Sum  Inputs=|++
  Sum1 : Sum  Inputs=|++
  out11 : Outport
  out12 : Outport  Port=2
  out21 : Outport  Port=3
  out22 : Outport  Port=4
  wires:
  K1_1/1 -> Gain1/1
  dtheta1/1 -> Product/2, Product1/2
  K1_2/1 -> Gain2/1
  dtheta2/1 -> Product2/2, Product3/2
  Gain1/1 -> Product/1, Product2/1
  Gain2/1 -> Product1/1, Product3/1
  Product/1 -> Sum/1
  SR/1 -> Sum/2, Sum1/2
  Product3/1 -> Sum1/1
  Sum/1 -> out11/1
  Product2/1 -> out12/1
  Product1/1 -> out21/1
  Sum1/1 -> out22/1

== system sus/RLS/P1/MATH1 ==
  note: (I - K*dtheta')*P
  in11 : Inport
  in12 : Inport  Port=2
  in21 : Inport  Port=3
  in22 : Inport  Port=4
  P11 : Inport  Port=5
  P12 : Inport  Port=6
  P21 : Inport  Port=7
  P22 : Inport  Port=8
  Product{,4..10} (8 alike) : Product  RndMeth=Zero
  Sum{,2..4} (4 alike) : Sum  Inputs=|++
  outP11 : Outport
  outP12 : Outport  Port=2
  outP21 : Outport  Port=3
  outP22 : Outport  Port=4
  wires:
  in11/1 -> Product/1, Product7/1
  in21/1 -> Product4/1, Product8/1
  in12/1 -> Product5/1, Product9/1
  in22/1 -> Product6/1, Product10/1
  Product/1 -> Sum/1
  Product5/1 -> Sum/2
  P11/1 -> Product/2, Product4/2
  P21/1 -> Product5/2, Product6/2
  Product4/1 -> Sum2/1
  Product6/1 -> Sum2/2
  Sum/1 -> outP11/1
  Sum2/1 -> outP21/1
  Product7/1 -> Sum3/1
  Product9/1 -> Sum3/2
  P12/1 -> Product7/2, Product8/2
  P22/1 -> Product9/2, Product10/2
  Product8/1 -> Sum4/1
  Product10/1 -> Sum4/2
  Sum4/1 -> outP22/1
  Sum3/1 -> outP12/1

== system sus/RLS/P2/HOLD ==
  In1 : Inport
  time : Inport  Port=2
  delay_in : Inport  Port=3
  CONST1 : Constant  Value=0
  CONST2 : Constant  Value=0
  Choice1 : Switch  Threshold=0.5-(1/16384)
  Choice2 : Switch  Threshold=0.5-(1/16384)
  Gain1 : Gain
  Gain2 : Gain  Gain=-1
  Sum8 : Sum  Inputs=+++
  out : Outport
  delay_out : Outport  Port=2
  wires:
  CONST2/1 -> Choice2/3
  time/1 -> Choice2/2, Choice1/2
  In1/1 -> Choice2/1
  Choice2/1 -> Sum8/2
  Sum8/1 -> delay_out/1
  delay_in/1 -> Gain2/1, Sum8/3, Gain1/1
  CONST1/1 -> Choice1/3
  Gain2/1 -> Choice1/1
  Choice1/1 -> Sum8/1
  Gain1/1 -> out/1

== system sus/RLS/P2/HOLD1 ==
  In1 : Inport
  time : Inport  Port=2
  delay_in : Inport  Port=3
  CONST1 : Constant  Value=0
  CONST2 : Constant  Value=0
  Choice1 : Switch  Threshold=0.5-(1/16384)
  Choice2 : Switch  Threshold=0.5-(1/16384)
  Gain1 : Gain
  Gain2 : Gain  Gain=-1
  Sum8 : Sum  Inputs=+++
  out : Outport
  delay_out : Outport  Port=2
  wires:
  CONST2/1 -> Choice2/3
  time/1 -> Choice2/2, Choice1/2
  In1/1 -> Choice2/1
  Choice2/1 -> Sum8/2
  Sum8/1 -> delay_out/1
  delay_in/1 -> Gain2/1, Sum8/3, Gain1/1
  CONST1/1 -> Choice1/3
  Gain2/1 -> Choice1/1
  Choice1/1 -> Sum8/1
  Gain1/1 -> out/1

== system sus/RLS/P2/HOLD2 ==
  In1 : Inport
  time : Inport  Port=2
  delay_in : Inport  Port=3
  CONST1 : Constant  Value=0
  CONST2 : Constant  Value=0
  Choice1 : Switch  Threshold=0.5-(1/16384)
  Choice2 : Switch  Threshold=0.5-(1/16384)
  Gain1 : Gain
  Gain2 : Gain  Gain=-1
  Sum8 : Sum  Inputs=+++
  out : Outport
  delay_out : Outport  Port=2
  wires:
  CONST2/1 -> Choice2/3
  time/1 -> Choice2/2, Choice1/2
  In1/1 -> Choice2/1
  Choice2/1 -> Sum8/2
  Sum8/1 -> delay_out/1
  delay_in/1 -> Gain2/1, Sum8/3, Gain1/1
  CONST1/1 -> Choice1/3
  Gain2/1 -> Choice1/1
  Choice1/1 -> Sum8/1
  Gain1/1 -> out/1

== system sus/RLS/P2/HOLD3 ==
  In1 : Inport
  time : Inport  Port=2
  delay_in : Inport  Port=3
  CONST1 : Constant  Value=0
  CONST2 : Constant  Value=0
  Choice1 : Switch  Threshold=0.5-(1/16384)
  Choice2 : Switch  Threshold=0.5-(1/16384)
  Gain1 : Gain
  Gain2 : Gain  Gain=-1
  Sum8 : Sum  Inputs=+++
  out : Outport
  delay_out : Outport  Port=2
  wires:
  CONST2/1 -> Choice2/3
  time/1 -> Choice2/2, Choice1/2
  In1/1 -> Choice2/1
  Choice2/1 -> Sum8/2
  Sum8/1 -> delay_out/1
  delay_in/1 -> Gain2/1, Sum8/3, Gain1/1
  CONST1/1 -> Choice1/3
  Gain2/1 -> Choice1/1
  Choice1/1 -> Sum8/1
  Gain1/1 -> out/1

== system sus/RLS/P2/MATH ==
  note: I - K*dtheta'
  K1_1 : Inport
  K1_2 : Inport  Port=2
  dtheta1 : Inport  Port=3
  dtheta2 : Inport  Port=4
  Gain1 : Gain  Gain=-1
  Gain2 : Gain  Gain=-1
  Product{,1..3} (4 alike) : Product  RndMeth=Zero
  SR : Constant
  Sum : Sum  Inputs=|++
  Sum1 : Sum  Inputs=|++
  out11 : Outport
  out12 : Outport  Port=2
  out21 : Outport  Port=3
  out22 : Outport  Port=4
  wires:
  K1_1/1 -> Gain1/1
  dtheta1/1 -> Product/2, Product1/2
  K1_2/1 -> Gain2/1
  dtheta2/1 -> Product2/2, Product3/2
  Gain1/1 -> Product/1, Product2/1
  Gain2/1 -> Product1/1, Product3/1
  Product/1 -> Sum/1
  SR/1 -> Sum/2, Sum1/2
  Product3/1 -> Sum1/1
  Sum/1 -> out11/1
  Product2/1 -> out12/1
  Product1/1 -> out21/1
  Sum1/1 -> out22/1

== system sus/RLS/P2/MATH1 ==
  note: (I - K*dtheta')*P
  in11 : Inport
  in12 : Inport  Port=2
  in21 : Inport  Port=3
  in22 : Inport  Port=4
  P11 : Inport  Port=5
  P12 : Inport  Port=6
  P21 : Inport  Port=7
  P22 : Inport  Port=8
  Product{,4..10} (8 alike) : Product  RndMeth=Zero
  Sum{,2..4} (4 alike) : Sum  Inputs=|++
  outP11 : Outport
  outP12 : Outport  Port=2
  outP21 : Outport  Port=3
  outP22 : Outport  Port=4
  wires:
  in11/1 -> Product/1, Product7/1
  in21/1 -> Product4/1, Product8/1
  in12/1 -> Product5/1, Product9/1
  in22/1 -> Product6/1, Product10/1
  Product/1 -> Sum/1
  Product5/1 -> Sum/2
  P11/1 -> Product/2, Product4/2
  P21/1 -> Product5/2, Product6/2
  Product4/1 -> Sum2/1
  Product6/1 -> Sum2/2
  Sum/1 -> outP11/1
  Sum2/1 -> outP21/1
  Product7/1 -> Sum3/1
  Product9/1 -> Sum3/2
  P12/1 -> Product7/2, Product8/2
  P22/1 -> Product9/2, Product10/2
  Product8/1 -> Sum4/1
  Product10/1 -> Sum4/2
  Sum4/1 -> outP22/1
  Sum3/1 -> outP12/1

== system sus/RLS/P3/HOLD ==
  In1 : Inport
  time : Inport  Port=2
  delay_in : Inport  Port=3
  CONST1 : Constant  Value=0
  CONST2 : Constant  Value=0
  Choice1 : Switch  Threshold=0.5-(1/16384)
  Choice2 : Switch  Threshold=0.5-(1/16384)
  Gain1 : Gain
  Gain2 : Gain  Gain=-1
  Sum8 : Sum  Inputs=+++
  out : Outport
  delay_out : Outport  Port=2
  wires:
  CONST2/1 -> Choice2/3
  time/1 -> Choice2/2, Choice1/2
  In1/1 -> Choice2/1
  Choice2/1 -> Sum8/2
  Sum8/1 -> delay_out/1
  delay_in/1 -> Gain2/1, Sum8/3, Gain1/1
  CONST1/1 -> Choice1/3
  Gain2/1 -> Choice1/1
  Choice1/1 -> Sum8/1
  Gain1/1 -> out/1

== system sus/RLS/P3/HOLD1 ==
  In1 : Inport
  time : Inport  Port=2
  delay_in : Inport  Port=3
  CONST1 : Constant  Value=0
  CONST2 : Constant  Value=0
  Choice1 : Switch  Threshold=0.5-(1/16384)
  Choice2 : Switch  Threshold=0.5-(1/16384)
  Gain1 : Gain
  Gain2 : Gain  Gain=-1
  Sum8 : Sum  Inputs=+++
  out : Outport
  delay_out : Outport  Port=2
  wires:
  CONST2/1 -> Choice2/3
  time/1 -> Choice2/2, Choice1/2
  In1/1 -> Choice2/1
  Choice2/1 -> Sum8/2
  Sum8/1 -> delay_out/1
  delay_in/1 -> Gain2/1, Sum8/3, Gain1/1
  CONST1/1 -> Choice1/3
  Gain2/1 -> Choice1/1
  Choice1/1 -> Sum8/1
  Gain1/1 -> out/1

== system sus/RLS/P3/HOLD2 ==
  In1 : Inport
  time : Inport  Port=2
  delay_in : Inport  Port=3
  CONST1 : Constant  Value=0
  CONST2 : Constant  Value=0
  Choice1 : Switch  Threshold=0.5-(1/16384)
  Choice2 : Switch  Threshold=0.5-(1/16384)
  Gain1 : Gain
  Gain2 : Gain  Gain=-1
  Sum8 : Sum  Inputs=+++
  out : Outport
  delay_out : Outport  Port=2
  wires:
  CONST2/1 -> Choice2/3
  time/1 -> Choice2/2, Choice1/2
  In1/1 -> Choice2/1
  Choice2/1 -> Sum8/2
  Sum8/1 -> delay_out/1
  delay_in/1 -> Gain2/1, Sum8/3, Gain1/1
  CONST1/1 -> Choice1/3
  Gain2/1 -> Choice1/1
  Choice1/1 -> Sum8/1
  Gain1/1 -> out/1

== system sus/RLS/P3/HOLD3 ==
  In1 : Inport
  time : Inport  Port=2
  delay_in : Inport  Port=3
  CONST1 : Constant  Value=0
  CONST2 : Constant  Value=0
  Choice1 : Switch  Threshold=0.5-(1/16384)
  Choice2 : Switch  Threshold=0.5-(1/16384)
  Gain1 : Gain
  Gain2 : Gain  Gain=-1
  Sum8 : Sum  Inputs=+++
  out : Outport
  delay_out : Outport  Port=2
  wires:
  CONST2/1 -> Choice2/3
  time/1 -> Choice2/2, Choice1/2
  In1/1 -> Choice2/1
  Choice2/1 -> Sum8/2
  Sum8/1 -> delay_out/1
  delay_in/1 -> Gain2/1, Sum8/3, Gain1/1
  CONST1/1 -> Choice1/3
  Gain2/1 -> Choice1/1
  Choice1/1 -> Sum8/1
  Gain1/1 -> out/1

== system sus/RLS/P3/MATH ==
  note: I - K*dtheta'
  K1_1 : Inport
  K1_2 : Inport  Port=2
  dtheta1 : Inport  Port=3
  dtheta2 : Inport  Port=4
  Gain1 : Gain  Gain=-1
  Gain2 : Gain  Gain=-1
  Product{,1..3} (4 alike) : Product  RndMeth=Zero
  SR : Constant
  Sum : Sum  Inputs=|++
  Sum1 : Sum  Inputs=|++
  out11 : Outport
  out12 : Outport  Port=2
  out21 : Outport  Port=3
  out22 : Outport  Port=4
  wires:
  K1_1/1 -> Gain1/1
  dtheta1/1 -> Product/2, Product1/2
  K1_2/1 -> Gain2/1
  dtheta2/1 -> Product2/2, Product3/2
  Gain1/1 -> Product/1, Product2/1
  Gain2/1 -> Product1/1, Product3/1
  Product/1 -> Sum/1
  SR/1 -> Sum/2, Sum1/2
  Product3/1 -> Sum1/1
  Sum/1 -> out11/1
  Product2/1 -> out12/1
  Product1/1 -> out21/1
  Sum1/1 -> out22/1

== system sus/RLS/P3/MATH1 ==
  note: (I - K*dtheta')*P
  in11 : Inport
  in12 : Inport  Port=2
  in21 : Inport  Port=3
  in22 : Inport  Port=4
  P11 : Inport  Port=5
  P12 : Inport  Port=6
  P21 : Inport  Port=7
  P22 : Inport  Port=8
  Product{,4..10} (8 alike) : Product  RndMeth=Zero
  Sum{,2..4} (4 alike) : Sum  Inputs=|++
  outP11 : Outport
  outP12 : Outport  Port=2
  outP21 : Outport  Port=3
  outP22 : Outport  Port=4
  wires:
  in11/1 -> Product/1, Product7/1
  in21/1 -> Product4/1, Product8/1
  in12/1 -> Product5/1, Product9/1
  in22/1 -> Product6/1, Product10/1
  Product/1 -> Sum/1
  Product5/1 -> Sum/2
  P11/1 -> Product/2, Product4/2
  P21/1 -> Product5/2, Product6/2
  Product4/1 -> Sum2/1
  Product6/1 -> Sum2/2
  Sum/1 -> outP11/1
  Sum2/1 -> outP21/1
  Product7/1 -> Sum3/1
  Product9/1 -> Sum3/2
  P12/1 -> Product7/2, Product8/2
  P22/1 -> Product9/2, Product10/2
  Product8/1 -> Sum4/1
  Product10/1 -> Sum4/2
  Sum4/1 -> outP22/1
  Sum3/1 -> outP12/1

== system sus/T1/E2S/SQRT_BOX1 ==
  In1 : Inport
  CONST11 : Constant  Value=0
  Choice : Switch  Threshold=1000
  Choice1 : Switch
  Choice2 : Switch  Threshold=1e10
  Choice3 : Switch  Threshold=0.01
  Choice4 : Switch  Threshold=1e-6
  Divide{,1..9} (10 alike) : Product  Inputs=*/  OutScaling=2^-10
  Gain : Gain  Gain=0.05
  Gain{1..10} (10 alike) : Gain  Gain=0.5
  Gain11 : Gain  Gain=0.0001
  Gain12 : Gain  Gain=0.000001
  Gain13 : Gain  Gain=100
  Gain14 : Gain  Gain=10000
  Sum{,1..9} (10 alike) : Sum  Inputs=|++
  Out1 : Outport
  wires:
  Divide/1 -> Sum/1
  Choice1/1 -> Choice/2, Choice2/2, Choice3/2, Choice4/2, Gain/1, Gain13/1, Gain14/1, Divide/1, Divide1/1, Divide2/1, Divide3/1, Divide4/1, Divide5/1, Divide6/1, Divide7/1, Divide8/1, Divide9/1, Gain12/1, Gain11/1
  Gain1/1 -> Sum1/2, Divide1/2
  Divide1/1 -> Sum1/1
  Sum1/1 -> Gain2/1
  Sum/1 -> Gain1/1
  Gain2/1 -> Sum2/2, Divide2/2
  Divide2/1 -> Sum2/1
  Sum2/1 -> Gain4/1
  Gain4/1 -> Sum3/2, Divide3/2
  Divide3/1 -> Sum3/1
  Sum3/1 -> Gain3/1
  Gain3/1 -> Sum4/2, Divide4/2
  Divide4/1 -> Sum4/1
  Sum4/1 -> Gain5/1
  Gain5/1 -> Sum5/2, Divide5/2
  Divide5/1 -> Sum5/1
  Sum5/1 -> Gain6/1
  Gain6/1 -> Sum6/2, Divide6/2
  Divide6/1 -> Sum6/1
  Sum6/1 -> Gain7/1
  Gain7/1 -> Sum7/2, Divide7/2
  Divide7/1 -> Sum7/1
  Sum7/1 -> Gain8/1
  Gain8/1 -> Sum8/2, Divide8/2
  Divide8/1 -> Sum8/1
  Sum8/1 -> Gain9/1
  Gain9/1 -> Sum9/2, Divide9/2
  Divide9/1 -> Sum9/1
  Sum9/1 -> Gain10/1
  Gain10/1 -> Out1/1
  Gain/1 -> Choice/3
  In1/1 -> Choice1/2, Choice1/1
  CONST11/1 -> Choice1/3
  Gain11/1 -> Choice2/3
  Gain12/1 -> Choice2/1
  Choice2/1 -> Choice/1
  Choice/1 -> Choice3/1
  Choice3/1 -> Choice4/1
  Choice4/1 -> Sum/2, Divide/2
  Gain13/1 -> Choice3/3
  Gain14/1 -> Choice4/3

== system sus/T1/E2S/SQRT_BOX2 ==
  In1 : Inport
  CONST11 : Constant  Value=0
  Choice : Switch  Threshold=1000
  Choice1 : Switch
  Choice2 : Switch  Threshold=1e10
  Choice3 : Switch  Threshold=0.01
  Choice4 : Switch  Threshold=1e-6
  Divide{,1..9} (10 alike) : Product  Inputs=*/  OutScaling=2^-10
  Gain : Gain  Gain=0.05
  Gain{1..10} (10 alike) : Gain  Gain=0.5
  Gain11 : Gain  Gain=0.0001
  Gain12 : Gain  Gain=0.000001
  Gain13 : Gain  Gain=100
  Gain14 : Gain  Gain=10000
  Sum{,1..9} (10 alike) : Sum  Inputs=|++
  Out1 : Outport
  wires:
  Divide/1 -> Sum/1
  Choice1/1 -> Choice/2, Choice2/2, Choice3/2, Choice4/2, Gain/1, Gain13/1, Gain14/1, Divide/1, Divide1/1, Divide2/1, Divide3/1, Divide4/1, Divide5/1, Divide6/1, Divide7/1, Divide8/1, Divide9/1, Gain12/1, Gain11/1
  Gain1/1 -> Sum1/2, Divide1/2
  Divide1/1 -> Sum1/1
  Sum1/1 -> Gain2/1
  Sum/1 -> Gain1/1
  Gain2/1 -> Sum2/2, Divide2/2
  Divide2/1 -> Sum2/1
  Sum2/1 -> Gain4/1
  Gain4/1 -> Sum3/2, Divide3/2
  Divide3/1 -> Sum3/1
  Sum3/1 -> Gain3/1
  Gain3/1 -> Sum4/2, Divide4/2
  Divide4/1 -> Sum4/1
  Sum4/1 -> Gain5/1
  Gain5/1 -> Sum5/2, Divide5/2
  Divide5/1 -> Sum5/1
  Sum5/1 -> Gain6/1
  Gain6/1 -> Sum6/2, Divide6/2
  Divide6/1 -> Sum6/1
  Sum6/1 -> Gain7/1
  Gain7/1 -> Sum7/2, Divide7/2
  Divide7/1 -> Sum7/1
  Sum7/1 -> Gain8/1
  Gain8/1 -> Sum8/2, Divide8/2
  Divide8/1 -> Sum8/1
  Sum8/1 -> Gain9/1
  Gain9/1 -> Sum9/2, Divide9/2
  Divide9/1 -> Sum9/1
  Sum9/1 -> Gain10/1
  Gain10/1 -> Out1/1
  Gain/1 -> Choice/3
  In1/1 -> Choice1/2, Choice1/1
  CONST11/1 -> Choice1/3
  Gain11/1 -> Choice2/3
  Gain12/1 -> Choice2/1
  Choice2/1 -> Choice/1
  Choice/1 -> Choice3/1
  Choice3/1 -> Choice4/1
  Choice4/1 -> Sum/2, Divide/2
  Gain13/1 -> Choice3/3
  Gain14/1 -> Choice4/3

== system sus/T1/E2S/SQRT_BOX3 ==
  In1 : Inport
  CONST11 : Constant  Value=0
  Choice : Switch  Threshold=1000
  Choice1 : Switch
  Choice2 : Switch  Threshold=1e10
  Choice3 : Switch  Threshold=0.01
  Choice4 : Switch  Threshold=1e-6
  Divide{,1..9} (10 alike) : Product  Inputs=*/  OutScaling=2^-10
  Gain : Gain  Gain=0.05
  Gain{1..10} (10 alike) : Gain  Gain=0.5
  Gain11 : Gain  Gain=0.0001
  Gain12 : Gain  Gain=0.000001
  Gain13 : Gain  Gain=100
  Gain14 : Gain  Gain=10000
  Sum{,1..9} (10 alike) : Sum  Inputs=|++
  Out1 : Outport
  wires:
  Divide/1 -> Sum/1
  Choice1/1 -> Choice/2, Choice2/2, Choice3/2, Choice4/2, Gain/1, Gain13/1, Gain14/1, Divide/1, Divide1/1, Divide2/1, Divide3/1, Divide4/1, Divide5/1, Divide6/1, Divide7/1, Divide8/1, Divide9/1, Gain12/1, Gain11/1
  Gain1/1 -> Sum1/2, Divide1/2
  Divide1/1 -> Sum1/1
  Sum1/1 -> Gain2/1
  Sum/1 -> Gain1/1
  Gain2/1 -> Sum2/2, Divide2/2
  Divide2/1 -> Sum2/1
  Sum2/1 -> Gain4/1
  Gain4/1 -> Sum3/2, Divide3/2
  Divide3/1 -> Sum3/1
  Sum3/1 -> Gain3/1
  Gain3/1 -> Sum4/2, Divide4/2
  Divide4/1 -> Sum4/1
  Sum4/1 -> Gain5/1
  Gain5/1 -> Sum5/2, Divide5/2
  Divide5/1 -> Sum5/1
  Sum5/1 -> Gain6/1
  Gain6/1 -> Sum6/2, Divide6/2
  Divide6/1 -> Sum6/1
  Sum6/1 -> Gain7/1
  Gain7/1 -> Sum7/2, Divide7/2
  Divide7/1 -> Sum7/1
  Sum7/1 -> Gain8/1
  Gain8/1 -> Sum8/2, Divide8/2
  Divide8/1 -> Sum8/1
  Sum8/1 -> Gain9/1
  Gain9/1 -> Sum9/2, Divide9/2
  Divide9/1 -> Sum9/1
  Sum9/1 -> Gain10/1
  Gain10/1 -> Out1/1
  Gain/1 -> Choice/3
  In1/1 -> Choice1/2, Choice1/1
  CONST11/1 -> Choice1/3
  Gain11/1 -> Choice2/3
  Gain12/1 -> Choice2/1
  Choice2/1 -> Choice/1
  Choice/1 -> Choice3/1
  Choice3/1 -> Choice4/1
  Choice4/1 -> Sum/2, Divide/2
  Gain13/1 -> Choice3/3
  Gain14/1 -> Choice4/3

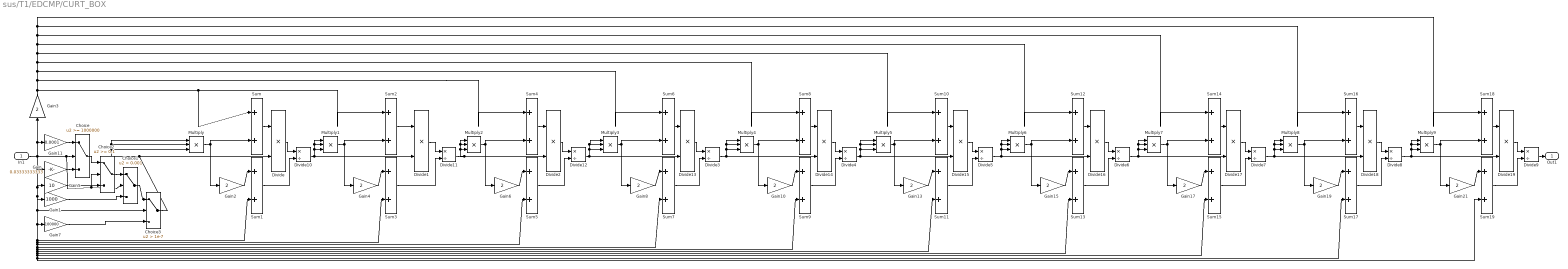
== system sus/T1/EDCMP/CURT_BOX ==
  In1 : Inport
  Choice : Switch  Threshold=1000000
  Choice1 : Switch  Criteria=u2 > Threshold  Threshold=0.001
  Choice2 : Switch  Threshold=0.1
  Choice3 : Switch  Criteria=u2 > Threshold  Threshold=1e-7
  Divide{,1..2,13..19} (10 alike) : Product  Inputs=**  OutScaling=2^-10
  Divide{3..12} (10 alike) : Product  Inputs=*/  OutScaling=2^-10
  Gain : Gain  Gain=0.03333333333
  Gain1 : Gain  Gain=1000
  Gain{2,4,6,8,10,13,15,17,19,21} (10 alike) : Gain  Gain=2
  Gain11 : Gain  Gain=0.0001
  Gain3 : Gain  Orientation=up  Gain=2
  Gain5 : Gain  Gain=10
  Gain7 : Gain  Gain=100000
  Multiply{,1..9} (10 alike) : Product  Inputs=***  OutScaling=2^-10
  Sum{,1..19} (20 alike) : Sum  Inputs=|++
  Out1 : Outport
  wires:
  In1/1 -> Gain/1, Gain1/1, Choice3/2, Sum1/2, Sum3/2, Sum5/2, Sum7/2, Sum9/2, Sum11/2, Sum13/2, Sum15/2, Sum17/2, Sum19/2, Gain7/1, Gain5/1, Choice/2, Choice2/2, Choice1/2, Gain11/1, Gain3/1
  Divide9/1 -> Out1/1
  Gain/1 -> Choice/3
  Gain11/1 -> Choice/1
  Choice3/1 -> Divide/2, Multiply/1, Multiply/2, Multiply/3
  Sum/1 -> Divide/1
  Multiply/1 -> Sum/2, Gain2/1
  Sum1/1 -> Divide10/2
  Gain2/1 -> Sum1/1
  Sum2/1 -> Divide1/1
  Multiply1/1 -> Sum2/2, Gain4/1
  Sum3/1 -> Divide11/2
  Gain4/1 -> Sum3/1
  Sum4/1 -> Divide2/1
  Multiply2/1 -> Sum4/2, Gain6/1
  Gain6/1 -> Sum5/1
  Divide12/1 -> Multiply3/1, Multiply3/2, Multiply3/3, Divide13/2
  Sum6/1 -> Divide13/1
  Multiply3/1 -> Sum6/2, Gain8/1
  Sum7/1 -> Divide3/2
  Gain8/1 -> Sum7/1
  Divide3/1 -> Multiply4/1, Multiply4/2, Multiply4/3, Divide14/2
  Sum8/1 -> Divide14/1
  Multiply4/1 -> Sum8/2, Gain10/1
  Sum9/1 -> Divide4/2
  Gain10/1 -> Sum9/1
  Divide4/1 -> Multiply5/1, Multiply5/2, Multiply5/3, Divide15/2
  Sum10/1 -> Divide15/1
  Multiply5/1 -> Sum10/2, Gain13/1
  Sum11/1 -> Divide5/2
  Gain13/1 -> Sum11/1
  Sum12/1 -> Divide16/1
  Multiply6/1 -> Sum12/2, Gain15/1
  Sum13/1 -> Divide6/2
  Gain15/1 -> Sum13/1
  Sum14/1 -> Divide17/1
  Multiply7/1 -> Sum14/2, Gain17/1
  Sum15/1 -> Divide7/2
  Gain17/1 -> Sum15/1
  Sum16/1 -> Divide18/1
  Multiply8/1 -> Sum16/2, Gain19/1
  Sum17/1 -> Divide8/2
  Gain19/1 -> Sum17/1
  Sum18/1 -> Divide19/1
  Multiply9/1 -> Sum18/2, Gain21/1
  Sum19/1 -> Divide9/2
  Gain21/1 -> Sum19/1
  Gain3/1 -> Sum16/1, Sum18/1, Sum14/1, Sum12/1, Sum10/1, Sum8/1, Sum6/1, Sum4/1, Sum2/1, Sum/1
  Divide/1 -> Divide10/1
  Divide10/1 -> Multiply1/1, Multiply1/2, Multiply1/3, Divide1/2
  Divide11/1 -> Divide2/2, Multiply2/1, Multiply2/2, Multiply2/3
  Divide1/1 -> Divide11/1
  Divide2/1 -> Divide12/1
  Sum5/1 -> Divide12/2
  Divide13/1 -> Divide3/1
  Divide14/1 -> Divide4/1
  Divide15/1 -> Divide5/1
  Divide5/1 -> Multiply6/1, Multiply6/2, Multiply6/3, Divide16/2
  Divide16/1 -> Divide6/1
  Divide6/1 -> Multiply7/1, Multiply7/2, Multiply7/3, Divide17/2
  Divide17/1 -> Divide7/1
  Divide7/1 -> Multiply8/1, Multiply8/2, Multiply8/3, Divide18/2
  Divide18/1 -> Divide8/1
  Divide8/1 -> Multiply9/1, Multiply9/2, Multiply9/3, Divide19/2
  Divide19/1 -> Divide9/1
  Gain1/1 -> Choice1/3
  Choice2/1 -> Choice1/1
  Choice/1 -> Choice2/1
  Gain5/1 -> Choice2/3
  Choice1/1 -> Choice3/1
  Gain7/1 -> Choice3/3
